simulink model "sdc_ut"  (Simulink 8.1)
settings: Solver=FixedStepDiscrete  StartTime=0.0  StopTime=Inf  FixedStep=0.005  RelTol=1e-3
PostLoadFcn:
  | , if any(exist('dsrtsu_mdlpostloadfcn', 'file') == [2, 3, 6]), try dsrtsu_mdlpostloadfcn('Execute', bdroot); catch fprintf('Error in PostLoadFcn (dsrtsu_mdlpostloadfcn) for model "%s":\n %s\n', bdroot, lasterr); end, end,
libraries: siltestlib x7, idiada_lib x7, sdc x1, hcu_lib x1
settings Model: DSRTSU_INTERNAL_RTI_VER=450  DSRTSU_INTERNAL_RTI_TYPE=rti1401  RTICANMMDATA=struct('GeneralSetupData',struct('modelroot','D:\ELN150201_TAIWAN\trunk\AdasDragon\software\sw_development\arch\app\ifo','generalsettings',struct('filesettings',struct('destfolder',struct('Name','RTICANMM_FILES','Check',1),'buildfolder',struct('Name','.','Check',1),'AbsDestfolder',struct('Name','D:\ELN150201_TAIWAN\trunk\AdasDragon\software\sw_development\arch\app\ifo\RTICANMM_FILES'),'AbsBuildfolder',struct('Name','D:\ELN150201_TAIWAN\trunk\AdasDragon\software\sw_development\arch\app\ifo'))),'options',struct('addpaths',1,'rmpaths',1,'addtrcexclusion',logical(1),'cannavigator',struct('checkmonitoring',0),'show_usrtrc',0,'use_usrtrc',0),'advanced',struct('options',[1 1 1 1 1 1 1 1 1 1 1 1 1 1 1 1 1 1 1 1 1 1 1 1 1 1 1 1 1 1 1 1 1 1 1 1 1 1 1 1 1 1 1 1 1 1 1 1 1 1 1 1 1 1 1 1 1 1 1 1 1 1 1 1 1 1 1 1 1 1 1 1 1 1 1 1 1 1 1 1 1 1 1 1 1 1 1 1 1 1 1 1 1 1 1 1 1 1 1 1]),'MPSetup',{{}},'modelname','sdc_ut','block','sdc_ut'))  DSRTSU_INTERNAL_RTIFPGA=40  Creator=tescamilla  LastModifiedBy=AT015555  BufferReuse=off
settings DataIOCC: SignalLoggingSaveFormat=Dataset
settings OptimizationCC: BlockReduction=off  OptimizeBlockIOStorage=off  BufferReuse=off  ExpressionFolding=off  ExpressionDepthLimit=128  LocalBlockOutputs=off
settings DebuggingCC: FcnCallInpInsideContextMsg=EnableAllAsError
settings HardwareCC: ProdIntDivRoundTo=Zero  ProdEndianess=BigEndian  ProdHWDeviceType=Generic->Custom  TargetIntDivRoundTo=Zero  TargetEndianess=BigEndian  TargetHWDeviceType=Generic->Custom
settings RTWCC: SystemTargetFile=rti1401.tlc  MakeCommand=make_rti  TemplateMakefile=rti1401.tmf  Description=dSPACE DS1401 Hardware Platform  ProcessScript=rti1401_make_rtw_hook
settings STFCustomTargetCC: CodeReplacementLibrary=ANSI_C  ParMdlRefBuildCompliant=on  GeneratePreprocessorConditionals=Disable all  MatFileLogging=on  SystemTargetFile=rti1401.tlc
settings GRTTargetCC: CompOptLevelCompliant=off  ConcurrentExecutionCompliant=off  ExtModeMexFile=noextcomm
settings CustomProperty: DataType=RTWOptions_EnumType_C__Program Files (x86)_dSPACE RCPHIL 2014-B_MATLAB_RTI_RTI1401_TLC_rti1401_1InitialSimState  Value=RUN
settings EnumStrPairs: String=RUN

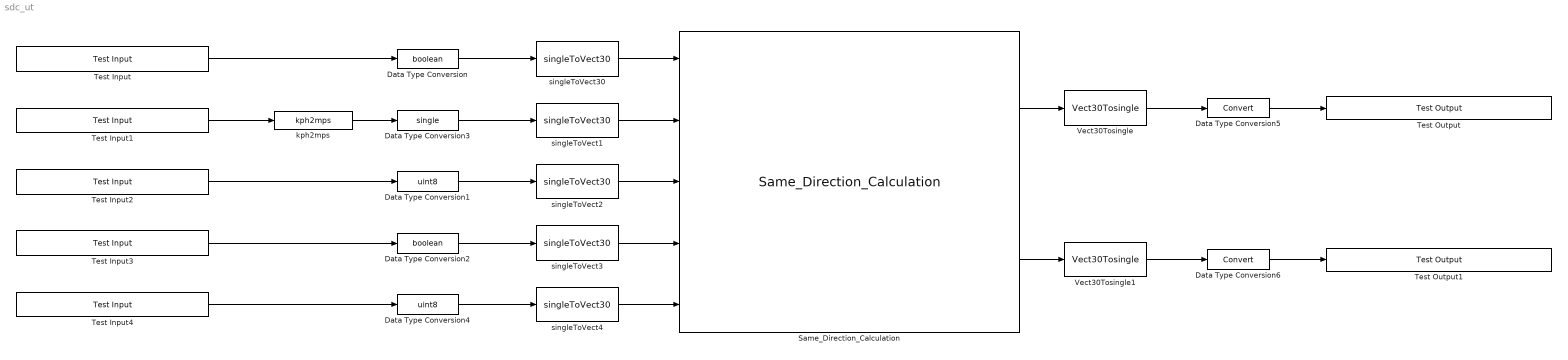
== system sdc_ut ==
  Data Type Conversion : DataTypeConversion  OutDataTypeStr=boolean
  Data Type Conversion1 : DataTypeConversion  OutDataTypeStr=uint8
  Data Type Conversion2 : DataTypeConversion  OutDataTypeStr=boolean
  Data Type Conversion3 : DataTypeConversion  OutDataTypeStr=single
  Data Type Conversion4 : DataTypeConversion  OutDataTypeStr=uint8
  Data Type Conversion5 : DataTypeConversion
  Data Type Conversion6 : DataTypeConversion
  Same_Direction_Calculation : sdc/Same_Direction_Calculation
  Test Input : siltestlib/Test Input  varname=VPER_RadObjValid_flg  sampletime=0.005
  Test Input1 : siltestlib/Test Input  varname=VIFO_TargAbsSpeedX_mps  sampletime=0.005
  Test Input2 : siltestlib/Test Input  varname=VPER_RadDynProperty_enum  sampletime=0.005
  Test Input3 : siltestlib/Test Input  varname=VPER_CamObstValid_flg  sampletime=0.005
  Test Input4 : siltestlib/Test Input  varname=VPER_CamObsStatus_enum  sampletime=0.005
  Test Output : siltestlib/Test Output  varname=VIFO_AEBSameDirectionVect30_flg  sampletime=-1
  Test Output1 : siltestlib/Test Output  varname=VIFO_ACCSameDirectionVect30_flg  sampletime=-1
  Vect30Tosingle : idiada_lib/Vect30Tosingle
  Vect30Tosingle1 : idiada_lib/Vect30Tosingle
  kph2mps : hcu_lib/kph2mps
  singleToVect{1..4,30} (5 alike) : idiada_lib/singleToVect30
  wires:
  Test Input/1 -> Data Type Conversion/1
  Data Type Conversion/1 -> singleToVect30/1
  Test Input1/1 -> kph2mps/1
  Data Type Conversion3/1 -> singleToVect1/1
  Test Input2/1 -> Data Type Conversion1/1
  Data Type Conversion1/1 -> singleToVect2/1
  Test Input3/1 -> Data Type Conversion2/1
  Data Type Conversion2/1 -> singleToVect3/1
  Test Input4/1 -> Data Type Conversion4/1
  Data Type Conversion4/1 -> singleToVect4/1
  Same_Direction_Calculation/1 -> Vect30Tosingle/1
  Data Type Conversion5/1 -> Test Output/1
  singleToVect30/1 -> Same_Direction_Calculation/1
  singleToVect1/1 -> Same_Direction_Calculation/2
  singleToVect2/1 -> Same_Direction_Calculation/3
  singleToVect3/1 -> Same_Direction_Calculation/4
  singleToVect4/1 -> Same_Direction_Calculation/5
  Vect30Tosingle/1 -> Data Type Conversion5/1
  kph2mps/1 -> Data Type Conversion3/1
  Same_Direction_Calculation/2 -> Vect30Tosingle1/1
  Data Type Conversion6/1 -> Test Output1/1
  Vect30Tosingle1/1 -> Data Type Conversion6/1
